simulink model "nonlinear_model"  (R2022a)
settings: Solver=VariableStepAuto  StartTime=0.0  StopTime=50  MaxStep=1e-3  RelTol=1e-3
values from neighbouring files (symbols this model uses):
  alfa1 = w0^2    (= 27.857284)    [approx_linear.m]    (also in nonlinear_file.m; trova_autovettori.m; trova_equilibri.m)
  alfa3 = -1.402*w0^2    (= -39.055912168)    [approx_linear.m]    (also in nonlinear_file.m; trova_autovettori.m; trova_equilibri.m)
  alfa5 = 0.271*w0^2    (= 7.549323964)    [approx_linear.m]    (also in nonlinear_file.m; trova_autovettori.m; trova_equilibri.m)
  mu1 = 0.086    [approx_linear.m]    (also in nonlinear_file.m; trova_autovettori.m; trova_equilibri.m)
  mu3 = 0.1080    (= 0.108)    [approx_linear.m]    (also in nonlinear_file.m; trova_autovettori.m; trova_equilibri.m)
settings Model: Creator=user  LastModifiedBy=user

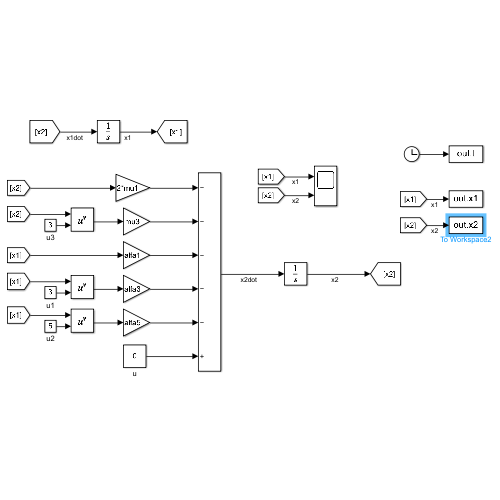
[thumbnail: Simulink's stored preview of the top-level diagram]
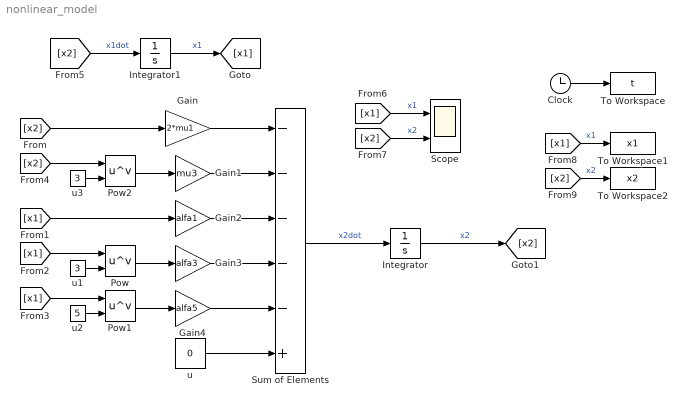
== system nonlinear_model ==
  Clock : Clock
  Gain : Gain  Gain=2*mu1
  Gain1 : Gain  Gain=mu3
  Gain2 : Gain  Gain=alfa1
  Gain3 : Gain  Gain=alfa3
  Gain4 : Gain  Gain=alfa5
  Integrator : Integrator  InitialCondition=0.5
  Integrator1 : Integrator  InitialCondition=0.5
  Pow : Math  Operator=pow  RndMeth=Zero
  Pow1 : Math  Operator=pow  RndMeth=Zero
  Pow2 : Math  Operator=pow  RndMeth=Zero
  Scope : Scope  NumInputPorts=2
  Sum of Elements : Sum  Inputs=-----+
  To Workspace : ToWorkspace  VariableName=t  SampleTime=-1
      settings: Save2DSignal=2-D array (concatenate along first dimension)
  To Workspace1 : ToWorkspace  VariableName=x1  SampleTime=-1
      settings: Save2DSignal=2-D array (concatenate along first dimension)
  To Workspace2 : ToWorkspace  VariableName=x2  SampleTime=-1
      settings: Save2DSignal=2-D array (concatenate along first dimension)
  u : Constant  Value=0
  u1 : Constant  Value=3
  u2 : Constant  Value=5
  u3 : Constant  Value=3
  wires:
  Gain1/1 -> Sum of Elements/2
  Gain/1 -> Sum of Elements/1
  Gain2/1 -> Sum of Elements/3
  Gain3/1 -> Sum of Elements/4
  Gain4/1 -> Sum of Elements/5
  u/1 -> Sum of Elements/6
  Sum of Elements/1 -> Integrator/1  "x2dot"
  Pow2/1 -> Gain1/1
  Pow/1 -> Gain3/1
  Pow1/1 -> Gain4/1
  [x1] -> Gain2/1
  [x1] -> Pow/1
  u1/1 -> Pow/2
  u2/1 -> Pow1/2
  [x1] -> Pow1/1
  Integrator/1 -> [x2]  "x2"
  [x2] -> Gain/1
  u3/1 -> Pow2/2
  [x2] -> Pow2/1
  [x2] -> Integrator1/1  "x1dot"
  Integrator1/1 -> [x1]  "x1"
  [x1] -> Scope/1  "x1"
  [x2] -> Scope/2  "x2"
  Clock/1 -> To Workspace/1
  [x1] -> To Workspace1/1  "x1"
  [x2] -> To Workspace2/1  "x2"
